simulink model "bh_4dof_LAGR_manipulator_CONTROL_DL_discrete"  (R2016b)
settings: Solver=ode23s  StartTime=0.0  StopTime=60  FixedStep=0.001  RelTol=1e-5  EnableMultiTasking=on
StopFcn:
  | bh_4dof_sim_post_process
values from neighbouring files (symbols this model uses):
  N = 3    [bh_4dof_sim_post_process.m]
undefined symbols (not defined in the file or in its folder): b1_damp, b2_damp, b3_damp, b4_damp, g, Hz, L1x, L1y, L1z, L2x, L2y, L2z, L3x, L3y, L3z, mass1, mass2, mass3, mass4, Rturn, theta1_0, theta1_dot_0, theta2_0, theta2_dot_0, theta3_0, theta3_dot_0, theta4_0, theta4_dot_0, X, Y, Z
libraries: simulink_extras x42, sm_lib x25, simulink x18, nesl_utility x17, discretizing x8
(part 1 of 4)
settings Model: Creator=bhorton  LastModifiedBy=bhorton
settings SolverCC: ZeroCrossAlgorithm=Adaptive
settings OptimizationCC: LifeSpan=inf
settings DebuggingCC: SFUnexpectedBacktrackingDiag=warning  SFNoUnconditionalDefaultTransitionDiag=warning  SFExecutionAtInitializationDiag=none
settings GRTTargetCC: TargetLangStandard=C89/C90 (ANSI)
settings ConfigComp: CovMetricSettings=dw  CovHtmlReporting=on  CovSaveCumulativeToWorkspaceVar=on  CovSaveSingleToWorkspaceVar=on  CovExternalEMLEnable=off
settings SimscapeCC: SimscapeLogDataHistory=10000  SelectedTab=General

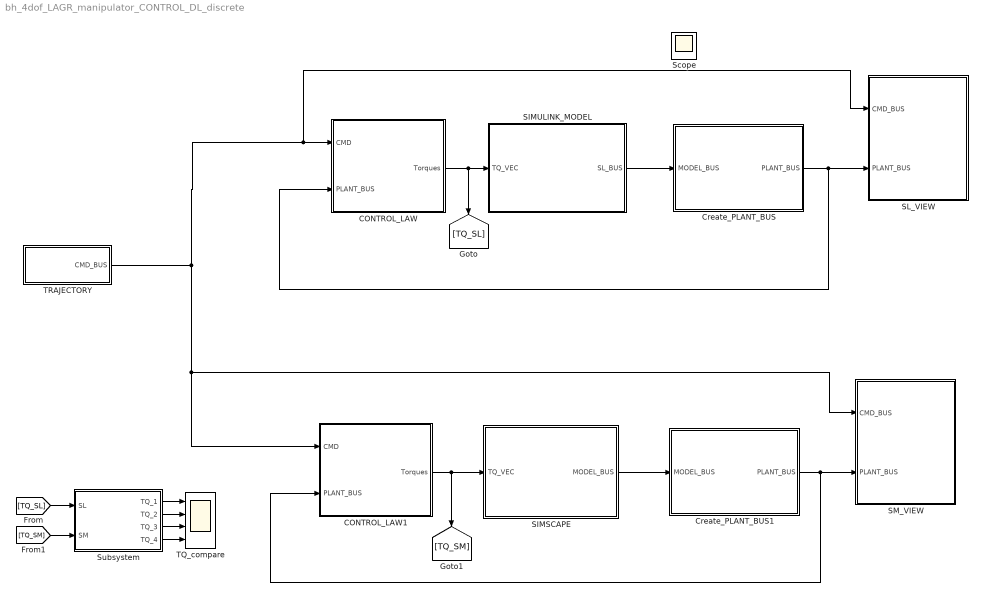
== system bh_4dof_LAGR_manipulator_CONTROL_DL_discrete ==
  CONTROL_LAW : Subsystem
  CONTROL_LAW1 : Subsystem
  Create_PLANT_BUS : Subsystem
  Create_PLANT_BUS1 : Subsystem
  SIMSCAPE : Subsystem  VariantControl=Variant
  SIMULINK_MODEL : Subsystem
  SL_VIEW : Subsystem
  SM_VIEW : Subsystem
  Subsystem : Subsystem
  TQ_compare : Scope  NumInputPorts=4
  TRAJECTORY : Subsystem
  Scope : Scope
  wires:
  TRAJECTORY/1(CMD_BUS) -> SL_VIEW/1(CMD_BUS), CONTROL_LAW/1(CMD), CONTROL_LAW1/1(CMD), SM_VIEW/1(CMD_BUS)
  Create_PLANT_BUS/1(PLANT_BUS) -> SL_VIEW/2(PLANT_BUS), CONTROL_LAW/2(PLANT_BUS)
  SIMULINK_MODEL/1(SL_BUS) -> Create_PLANT_BUS/1(MODEL_BUS)
  CONTROL_LAW/1(Torques) -> SIMULINK_MODEL/1(TQ_VEC), [TQ_SL]
  SIMSCAPE/1(MODEL_BUS) -> Create_PLANT_BUS1/1(MODEL_BUS)
  CONTROL_LAW1/1(Torques) -> SIMSCAPE/1(TQ_VEC), [TQ_SM]
  Create_PLANT_BUS1/1(PLANT_BUS) -> CONTROL_LAW1/2(PLANT_BUS), SM_VIEW/2(PLANT_BUS)
  [TQ_SL] -> Subsystem/1(SL)
  [TQ_SM] -> Subsystem/2(SM)
  Subsystem/1(TQ_1) -> TQ_compare/1
  Subsystem/4(TQ_4) -> TQ_compare/4
  Subsystem/2(TQ_2) -> TQ_compare/2
  Subsystem/3(TQ_3) -> TQ_compare/3

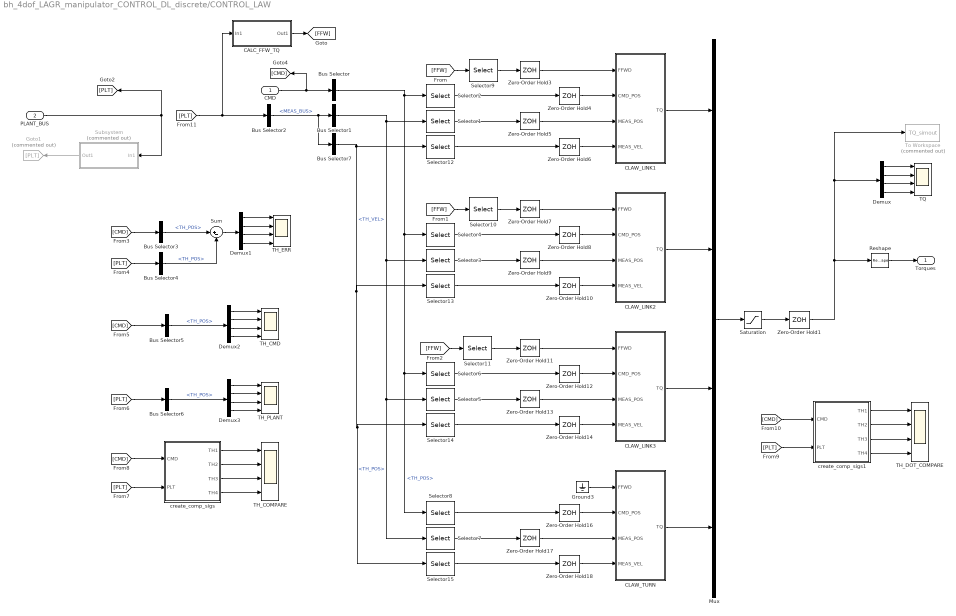
== system bh_4dof_LAGR_manipulator_CONTROL_DL_discrete/CONTROL_LAW ==
  CMD : Inport
  PLANT_BUS : Inport  Port=2
  Bus Selector{,1,3,5} (4 alike) : BusSelector  OutputSignals=TH_POS
  Bus Selector2 : BusSelector  OutputSignals=MEAS_BUS
  Bus Selector4 : BusSelector  OutputSignals=MEAS_BUS.TH_POS
  Bus Selector6 : BusSelector  OutputSignals=MEAS_BUS.TH_POS
  Bus Selector7 : BusSelector  OutputSignals=TH_VEL
  CALC_FFW_TQ : Subsystem
  CLAW_LINK1 : Subsystem
  CLAW_LINK2 : Subsystem
  CLAW_LINK3 : Subsystem
  CLAW_TURN : Subsystem
  Demux{,1..3} (4 alike) : Demux
  Goto1 : Goto  Commented=on  GotoTag=PLT
  Ground3 : Ground
  Mux : Mux
  Reshape : Reshape  OutputDimensionality=Column vector (2-D)
  Saturation : Saturate  UpperLimit=3  LowerLimit=-3
  Selector1 : Selector  InputPortWidth=4  IndexOptions=Index vector (dialog)  Indices=1  OutputSizes=1
  Selector10 : Selector  InputPortWidth=3  IndexOptions=Index vector (dialog)  Indices=2  OutputSizes=1
  Selector11 : Selector  InputPortWidth=3  IndexOptions=Index vector (dialog)  Indices=3  OutputSizes=1
  Selector12 : Selector  InputPortWidth=4  IndexOptions=Index vector (dialog)  Indices=1  OutputSizes=1
  Selector13 : Selector  InputPortWidth=4  IndexOptions=Index vector (dialog)  Indices=2  OutputSizes=1
  Selector14 : Selector  InputPortWidth=4  IndexOptions=Index vector (dialog)  Indices=3  OutputSizes=1
  Selector15 : Selector  InputPortWidth=4  IndexOptions=Index vector (dialog)  Indices=4  OutputSizes=1
  Selector2 : Selector  InputPortWidth=4  IndexOptions=Index vector (dialog)  Indices=1  OutputSizes=1
  Selector3 : Selector  InputPortWidth=4  IndexOptions=Index vector (dialog)  Indices=2  OutputSizes=1
  Selector4 : Selector  InputPortWidth=4  IndexOptions=Index vector (dialog)  Indices=2  OutputSizes=1
  Selector5 : Selector  InputPortWidth=4  IndexOptions=Index vector (dialog)  Indices=3  OutputSizes=1
  Selector6 : Selector  InputPortWidth=4  IndexOptions=Index vector (dialog)  Indices=3  OutputSizes=1
  Selector7 : Selector  InputPortWidth=4  IndexOptions=Index vector (dialog)  Indices=4  OutputSizes=1
  Selector8 : Selector  InputPortWidth=4  IndexOptions=Index vector (dialog)  Indices=4  OutputSizes=1
  Selector9 : Selector  InputPortWidth=3  IndexOptions=Index vector (dialog)  Indices=1  OutputSizes=1
  Subsystem : Subsystem  Commented=on
  Sum : Sum  Inputs=|+-
  TH_CMD : Scope  NumInputPorts=4
  TH_COMPARE : Scope  NumInputPorts=4
  TH_DOT_COMPARE : Scope  NumInputPorts=4
  TH_ERR : Scope  NumInputPorts=4
  TH_PLANT : Scope  NumInputPorts=4
  TQ : Scope  NumInputPorts=4
  To Workspace : ToWorkspace  Commented=on  VariableName=TQ_simout  SaveFormat=Structure With Time  SampleTime=-1
  Zero-Order Hold{1,3..14,16..18} (16 alike) : ZeroOrderHold  SampleTime=0.001
      settings: AttributesFormatString=DT =%<SampleTime>
  create_comp_sigs : Subsystem
  create_comp_sigs1 : Subsystem
  Torques : Outport
  wires:
  Mux/1 -> Saturation/1
  Reshape/1 -> Torques/1
  Selector9/1 -> Zero-Order Hold3/1
  CMD/1 -> [CMD], Bus Selector/1
  Selector1/1 -> Zero-Order Hold5/1
  Selector2/1 -> Zero-Order Hold4/1
  Bus Selector/1 -> Selector8/1, Selector6/1, Selector4/1, Selector2/1  "<TH_POS>"
  Bus Selector1/1 -> Selector5/1, Selector7/1, Selector3/1, Selector1/1  "<TH_POS>"
  Bus Selector2/1 -> Bus Selector7/1, Bus Selector1/1  "<MEAS_BUS>"
  Demux/1 -> TQ/1
  Demux/2 -> TQ/2
  Demux/4 -> TQ/4
  Demux/3 -> TQ/3
  CALC_FFW_TQ/1(Out1) -> [FFW]
  [FFW] -> Selector9/1
  [FFW] -> Selector10/1
  [FFW] -> Selector11/1
  Demux1/1 -> TH_ERR/1
  Demux1/2 -> TH_ERR/2
  Demux1/4 -> TH_ERR/4
  Demux1/3 -> TH_ERR/3
  PLANT_BUS/1 -> Subsystem/1(In1), [PLT]
  [CMD] -> Bus Selector3/1
  [PLT] -> Bus Selector4/1
  Bus Selector3/1 -> Sum/1  "<TH_POS>"
  Bus Selector4/1 -> Sum/2  "<TH_POS>"
  Sum/1 -> Demux1/1
  Demux2/1 -> TH_CMD/1
  Demux2/2 -> TH_CMD/2
  Demux2/4 -> TH_CMD/4
  Demux2/3 -> TH_CMD/3
  [CMD] -> Bus Selector5/1
  Bus Selector5/1 -> Demux2/1  "<TH_POS>"
  Demux3/1 -> TH_PLANT/1
  Demux3/2 -> TH_PLANT/2
  Demux3/4 -> TH_PLANT/4
  Demux3/3 -> TH_PLANT/3
  [PLT] -> Bus Selector6/1
  Bus Selector6/1 -> Demux3/1  "<TH_POS>"
  Bus Selector7/1 -> Selector15/1, Selector14/1, Selector13/1, Selector12/1  "<TH_VEL>"
  Selector12/1 -> Zero-Order Hold6/1
  CLAW_TURN/1(TQ) -> Mux/4
  CLAW_LINK3/1(TQ) -> Mux/3
  CLAW_LINK2/1(TQ) -> Mux/2
  CLAW_LINK1/1(TQ) -> Mux/1
  Saturation/1 -> Zero-Order Hold1/1
  Zero-Order Hold3/1 -> CLAW_LINK1/1(FFWD)
  Zero-Order Hold4/1 -> CLAW_LINK1/2(CMD_POS)
  Zero-Order Hold5/1 -> CLAW_LINK1/3(MEAS_POS)
  Zero-Order Hold6/1 -> CLAW_LINK1/4(MEAS_VEL)
  Selector10/1 -> Zero-Order Hold7/1
  Selector3/1 -> Zero-Order Hold9/1
  Selector4/1 -> Zero-Order Hold8/1
  Selector13/1 -> Zero-Order Hold10/1
  Zero-Order Hold7/1 -> CLAW_LINK2/1(FFWD)
  Zero-Order Hold8/1 -> CLAW_LINK2/2(CMD_POS)
  Zero-Order Hold9/1 -> CLAW_LINK2/3(MEAS_POS)
  Zero-Order Hold10/1 -> CLAW_LINK2/4(MEAS_VEL)
  Selector5/1 -> Zero-Order Hold13/1
  Selector6/1 -> Zero-Order Hold12/1
  Selector14/1 -> Zero-Order Hold14/1
  Zero-Order Hold11/1 -> CLAW_LINK3/1(FFWD)
  Zero-Order Hold12/1 -> CLAW_LINK3/2(CMD_POS)
  Zero-Order Hold13/1 -> CLAW_LINK3/3(MEAS_POS)
  Zero-Order Hold14/1 -> CLAW_LINK3/4(MEAS_VEL)
  Selector11/1 -> Zero-Order Hold11/1
  Selector7/1 -> Zero-Order Hold17/1
  Selector8/1 -> Zero-Order Hold16/1
  Selector15/1 -> Zero-Order Hold18/1
  Zero-Order Hold16/1 -> CLAW_TURN/2(CMD_POS)
  Zero-Order Hold17/1 -> CLAW_TURN/3(MEAS_POS)
  Zero-Order Hold18/1 -> CLAW_TURN/4(MEAS_VEL)
  Ground3/1 -> CLAW_TURN/1(FFWD)
  [PLT] -> create_comp_sigs/2(PLT)
  [CMD] -> create_comp_sigs/1(CMD)
  create_comp_sigs/1(TH1) -> TH_COMPARE/1
  create_comp_sigs/2(TH2) -> TH_COMPARE/2
  create_comp_sigs/3(TH3) -> TH_COMPARE/3
  create_comp_sigs/4(TH4) -> TH_COMPARE/4
  [PLT] -> create_comp_sigs1/2(PLT)
  [CMD] -> create_comp_sigs1/1(CMD)
  create_comp_sigs1/1(TH1) -> TH_DOT_COMPARE/1
  create_comp_sigs1/2(TH2) -> TH_DOT_COMPARE/2
  create_comp_sigs1/3(TH3) -> TH_DOT_COMPARE/3
  create_comp_sigs1/4(TH4) -> TH_DOT_COMPARE/4
  Zero-Order Hold1/1 -> Reshape/1, To Workspace/1, Demux/1
  Subsystem/1(Out1) -> Goto1/1
  [PLT] -> CALC_FFW_TQ/1(In1), Bus Selector2/1

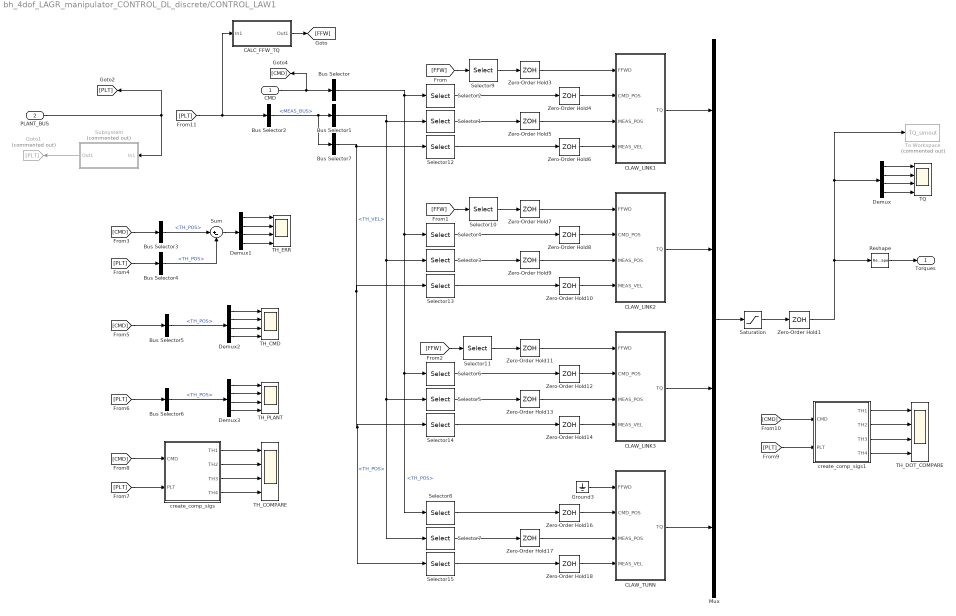
== system bh_4dof_LAGR_manipulator_CONTROL_DL_discrete/CONTROL_LAW1 ==
  CMD : Inport
  PLANT_BUS : Inport  Port=2
  Bus Selector{,1,3,5} (4 alike) : BusSelector  OutputSignals=TH_POS
  Bus Selector2 : BusSelector  OutputSignals=MEAS_BUS
  Bus Selector4 : BusSelector  OutputSignals=MEAS_BUS.TH_POS
  Bus Selector6 : BusSelector  OutputSignals=MEAS_BUS.TH_POS
  Bus Selector7 : BusSelector  OutputSignals=TH_VEL
  CALC_FFW_TQ : Subsystem
  CLAW_LINK1 : Subsystem
  CLAW_LINK2 : Subsystem
  CLAW_LINK3 : Subsystem
  CLAW_TURN : Subsystem
  Demux{,1..3} (4 alike) : Demux
  Goto1 : Goto  Commented=on  GotoTag=PLT
  Ground3 : Ground
  Mux : Mux
  Reshape : Reshape  OutputDimensionality=Column vector (2-D)
  Saturation : Saturate  UpperLimit=3  LowerLimit=-3
  Selector1 : Selector  InputPortWidth=4  IndexOptions=Index vector (dialog)  Indices=1  OutputSizes=1
  Selector10 : Selector  InputPortWidth=3  IndexOptions=Index vector (dialog)  Indices=2  OutputSizes=1
  Selector11 : Selector  InputPortWidth=3  IndexOptions=Index vector (dialog)  Indices=3  OutputSizes=1
  Selector12 : Selector  InputPortWidth=4  IndexOptions=Index vector (dialog)  Indices=1  OutputSizes=1
  Selector13 : Selector  InputPortWidth=4  IndexOptions=Index vector (dialog)  Indices=2  OutputSizes=1
  Selector14 : Selector  InputPortWidth=4  IndexOptions=Index vector (dialog)  Indices=3  OutputSizes=1
  Selector15 : Selector  InputPortWidth=4  IndexOptions=Index vector (dialog)  Indices=4  OutputSizes=1
  Selector2 : Selector  InputPortWidth=4  IndexOptions=Index vector (dialog)  Indices=1  OutputSizes=1
  Selector3 : Selector  InputPortWidth=4  IndexOptions=Index vector (dialog)  Indices=2  OutputSizes=1
  Selector4 : Selector  InputPortWidth=4  IndexOptions=Index vector (dialog)  Indices=2  OutputSizes=1
  Selector5 : Selector  InputPortWidth=4  IndexOptions=Index vector (dialog)  Indices=3  OutputSizes=1
  Selector6 : Selector  InputPortWidth=4  IndexOptions=Index vector (dialog)  Indices=3  OutputSizes=1
  Selector7 : Selector  InputPortWidth=4  IndexOptions=Index vector (dialog)  Indices=4  OutputSizes=1
  Selector8 : Selector  InputPortWidth=4  IndexOptions=Index vector (dialog)  Indices=4  OutputSizes=1
  Selector9 : Selector  InputPortWidth=3  IndexOptions=Index vector (dialog)  Indices=1  OutputSizes=1
  Subsystem : Subsystem  Commented=on
  Sum : Sum  Inputs=|+-
  TH_CMD : Scope  NumInputPorts=4
  TH_COMPARE : Scope  NumInputPorts=4
  TH_DOT_COMPARE : Scope  NumInputPorts=4
  TH_ERR : Scope  NumInputPorts=4
  TH_PLANT : Scope  NumInputPorts=4
  TQ : Scope  NumInputPorts=4
  To Workspace : ToWorkspace  Commented=on  VariableName=TQ_simout  SaveFormat=Structure With Time  SampleTime=-1
  Zero-Order Hold{1,3..14,16..18} (16 alike) : ZeroOrderHold  SampleTime=0.001
      settings: AttributesFormatString=DT =%<SampleTime>
  create_comp_sigs : Subsystem
  create_comp_sigs1 : Subsystem
  Torques : Outport
  wires:
  Mux/1 -> Saturation/1
  Reshape/1 -> Torques/1
  Selector9/1 -> Zero-Order Hold3/1
  CMD/1 -> [CMD], Bus Selector/1
  Selector1/1 -> Zero-Order Hold5/1
  Selector2/1 -> Zero-Order Hold4/1
  Bus Selector/1 -> Selector8/1, Selector6/1, Selector4/1, Selector2/1  "<TH_POS>"
  Bus Selector1/1 -> Selector5/1, Selector7/1, Selector3/1, Selector1/1  "<TH_POS>"
  Bus Selector2/1 -> Bus Selector7/1, Bus Selector1/1  "<MEAS_BUS>"
  Demux/1 -> TQ/1
  Demux/2 -> TQ/2
  Demux/4 -> TQ/4
  Demux/3 -> TQ/3
  CALC_FFW_TQ/1(Out1) -> [FFW]
  [FFW] -> Selector9/1
  [FFW] -> Selector10/1
  [FFW] -> Selector11/1
  Demux1/1 -> TH_ERR/1
  Demux1/2 -> TH_ERR/2
  Demux1/4 -> TH_ERR/4
  Demux1/3 -> TH_ERR/3
  PLANT_BUS/1 -> Subsystem/1(In1), [PLT]
  [CMD] -> Bus Selector3/1
  [PLT] -> Bus Selector4/1
  Bus Selector3/1 -> Sum/1  "<TH_POS>"
  Bus Selector4/1 -> Sum/2  "<TH_POS>"
  Sum/1 -> Demux1/1
  Demux2/1 -> TH_CMD/1
  Demux2/2 -> TH_CMD/2
  Demux2/4 -> TH_CMD/4
  Demux2/3 -> TH_CMD/3
  [CMD] -> Bus Selector5/1
  Bus Selector5/1 -> Demux2/1  "<TH_POS>"
  Demux3/1 -> TH_PLANT/1
  Demux3/2 -> TH_PLANT/2
  Demux3/4 -> TH_PLANT/4
  Demux3/3 -> TH_PLANT/3
  [PLT] -> Bus Selector6/1
  Bus Selector6/1 -> Demux3/1  "<TH_POS>"
  Bus Selector7/1 -> Selector15/1, Selector14/1, Selector13/1, Selector12/1  "<TH_VEL>"
  Selector12/1 -> Zero-Order Hold6/1
  CLAW_TURN/1(TQ) -> Mux/4
  CLAW_LINK3/1(TQ) -> Mux/3
  CLAW_LINK2/1(TQ) -> Mux/2
  CLAW_LINK1/1(TQ) -> Mux/1
  Saturation/1 -> Zero-Order Hold1/1
  Zero-Order Hold3/1 -> CLAW_LINK1/1(FFWD)
  Zero-Order Hold4/1 -> CLAW_LINK1/2(CMD_POS)
  Zero-Order Hold5/1 -> CLAW_LINK1/3(MEAS_POS)
  Zero-Order Hold6/1 -> CLAW_LINK1/4(MEAS_VEL)
  Selector10/1 -> Zero-Order Hold7/1
  Selector3/1 -> Zero-Order Hold9/1
  Selector4/1 -> Zero-Order Hold8/1
  Selector13/1 -> Zero-Order Hold10/1
  Zero-Order Hold7/1 -> CLAW_LINK2/1(FFWD)
  Zero-Order Hold8/1 -> CLAW_LINK2/2(CMD_POS)
  Zero-Order Hold9/1 -> CLAW_LINK2/3(MEAS_POS)
  Zero-Order Hold10/1 -> CLAW_LINK2/4(MEAS_VEL)
  Selector5/1 -> Zero-Order Hold13/1
  Selector6/1 -> Zero-Order Hold12/1
  Selector14/1 -> Zero-Order Hold14/1
  Zero-Order Hold11/1 -> CLAW_LINK3/1(FFWD)
  Zero-Order Hold12/1 -> CLAW_LINK3/2(CMD_POS)
  Zero-Order Hold13/1 -> CLAW_LINK3/3(MEAS_POS)
  Zero-Order Hold14/1 -> CLAW_LINK3/4(MEAS_VEL)
  Selector11/1 -> Zero-Order Hold11/1
  Selector7/1 -> Zero-Order Hold17/1
  Selector8/1 -> Zero-Order Hold16/1
  Selector15/1 -> Zero-Order Hold18/1
  Zero-Order Hold16/1 -> CLAW_TURN/2(CMD_POS)
  Zero-Order Hold17/1 -> CLAW_TURN/3(MEAS_POS)
  Zero-Order Hold18/1 -> CLAW_TURN/4(MEAS_VEL)
  Ground3/1 -> CLAW_TURN/1(FFWD)
  [PLT] -> create_comp_sigs/2(PLT)
  [CMD] -> create_comp_sigs/1(CMD)
  create_comp_sigs/1(TH1) -> TH_COMPARE/1
  create_comp_sigs/2(TH2) -> TH_COMPARE/2
  create_comp_sigs/3(TH3) -> TH_COMPARE/3
  create_comp_sigs/4(TH4) -> TH_COMPARE/4
  [PLT] -> create_comp_sigs1/2(PLT)
  [CMD] -> create_comp_sigs1/1(CMD)
  create_comp_sigs1/1(TH1) -> TH_DOT_COMPARE/1
  create_comp_sigs1/2(TH2) -> TH_DOT_COMPARE/2
  create_comp_sigs1/3(TH3) -> TH_DOT_COMPARE/3
  create_comp_sigs1/4(TH4) -> TH_DOT_COMPARE/4
  Zero-Order Hold1/1 -> Reshape/1, To Workspace/1, Demux/1
  Subsystem/1(Out1) -> Goto1/1
  [PLT] -> CALC_FFW_TQ/1(In1), Bus Selector2/1

== system bh_4dof_LAGR_manipulator_CONTROL_DL_discrete/Create_PLANT_BUS ==
  MODEL_BUS : Inport
  CALC_BUS : Subsystem
  MEAS : Subsystem
  Subsystem : Subsystem
  Subsystem1 : Subsystem
  PLANT_BUS : Outport
  wires:
  MODEL_BUS/1 -> MEAS/1(MODEL_BUS), CALC_BUS/1(MODEL_BUS), Subsystem/1(MODEL)
  Subsystem/1(PLANT_B) -> PLANT_BUS/1
  CALC_BUS/1(CALC_POS) -> Subsystem1/1(POS), Subsystem/3(CALC_POS)
  MEAS/1(MEAS) -> Subsystem/2(MEAS)
  Subsystem1/1(GTQ) -> Subsystem/4(CALC_GRAV_TQ)

== system bh_4dof_LAGR_manipulator_CONTROL_DL_discrete/Create_PLANT_BUS1 ==
  MODEL_BUS : Inport
  CALC_BUS : Subsystem
  MEAS : Subsystem
  Subsystem : Subsystem
  Subsystem1 : Subsystem
  PLANT_BUS : Outport
  wires:
  MODEL_BUS/1 -> MEAS/1(MODEL_BUS), CALC_BUS/1(MODEL_BUS), Subsystem/1(MODEL)
  Subsystem/1(PLANT_B) -> PLANT_BUS/1
  CALC_BUS/1(CALC_POS) -> Subsystem1/1(POS), Subsystem/3(CALC_POS)
  MEAS/1(MEAS) -> Subsystem/2(MEAS)
  Subsystem1/1(GTQ) -> Subsystem/4(CALC_GRAV_TQ)

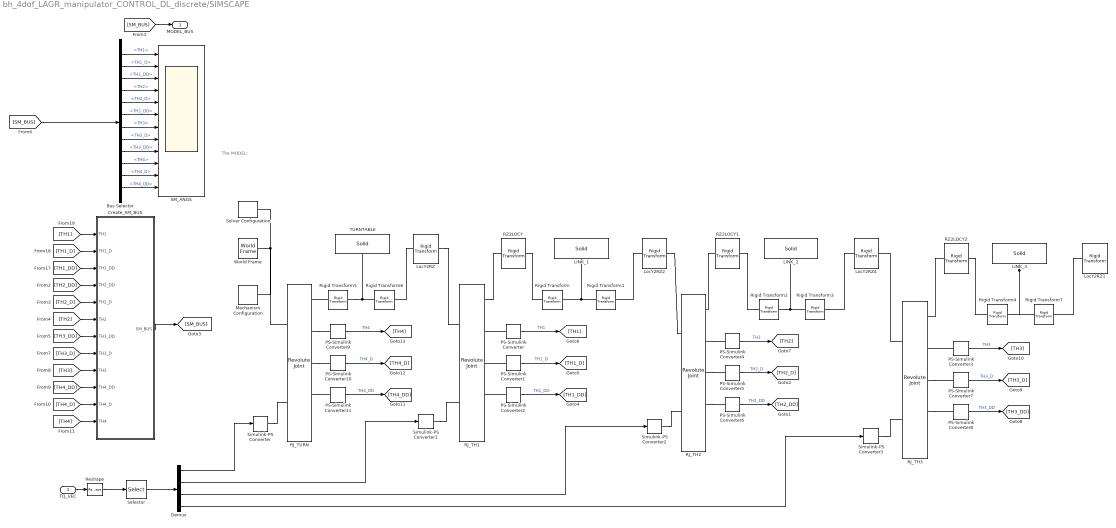
== system bh_4dof_LAGR_manipulator_CONTROL_DL_discrete/SIMSCAPE ==
  note: The MODEL:
  TQ_VEC : Inport
  Bus Selector : BusSelector  OutputSignals=TH1,TH1_D,TH1_DD,TH2,TH2_D,TH2_DD,TH3,TH3_D,TH3_DD,TH4,TH4_D,TH4_DD
  Create_SM_BUS : Subsystem
  Demux : Demux
  LINK_1 : sm_lib/Body Elements/Solid  InertiaType=CalculateFromGeometry  Mass=1  MassUnits=kg  CenterOfMass=[0 0 0]  CenterOfMassUnits=m  MomentsOfInertia=[1 1 1]  MomentsOfInertiaUnits=kg*m^2  ProductsOfInertia=[0 0 0]  ProductsOfInertiaUnits=kg*m^2  DensityBased=on  Density=density  DensityUnits=kg/(m^3)  DoExposeReferenceFrame=on  SerializedFrames=<Frames/>  GraphicType=FromGeometry  MarkerShape=Sphere  MarkerSize=10  GraphicVisPropType=SimpleVisualProperties  GraphicDiffuseColor=[0.2 0.2 1.0]  GraphicSpecularColor=[0.5 0.5 0.5 1.0]  GraphicAmbientColor=[0.15 0.15 0.15 1.0]  GraphicEmissiveColor=[0.0 0.0 0.0 1.0]  GraphicShininess=75  GraphicOpacity=1.0  GeometryShape=Brick  RectangleSize=[1 1]  RectangleSizeUnits=m  BrickDimensions=[L1x, L1y, L1z ]  BrickDimensionUnits=m  CylinderRadius=1  CylinderRadiusUnits=m  CylinderLength=1  CylinderLengthUnits=m  SphereRadius=1  SphereRadiusUnits=m  EllipsoidRadii=[1 1 1]  EllipsoidRadiiUnits=m  ExtrusionCrossSection=[1 1; -1 1; -1 -1; 1 -1]  ExtrusionCrossSectionUnits=m  ExtrusionLength=1  ExtrusionLengthUnits=m  PolygonNumSides=3  PolygonOuterRadius=1  PolygonOuterRadiusUnits=m  ExtGeomFileType=STEP  ExtGeomFileUnits=m  RevolutionCrossSection=[1 1; 1 -1; 2 -1; 2 1]  RevolutionCrossSectionUnits=m  RevolutionExtent=Full  RevolutionAngle=180  RevolutionAngleUnits=deg
  LINK_2 : sm_lib/Body Elements/Solid  InertiaType=CalculateFromGeometry  Mass=1  MassUnits=kg  CenterOfMass=[0 0 0]  CenterOfMassUnits=m  MomentsOfInertia=[1 1 1]  MomentsOfInertiaUnits=kg*m^2  ProductsOfInertia=[0 0 0]  ProductsOfInertiaUnits=kg*m^2  DensityBased=on  Density=density  DensityUnits=kg/(m^3)  DoExposeReferenceFrame=on  SerializedFrames=<Frames/>  GraphicType=FromGeometry  MarkerShape=Sphere  MarkerSize=10  GraphicVisPropType=SimpleVisualProperties  GraphicDiffuseColor=[0.8 0.8 1.0]  GraphicSpecularColor=[0.5 0.5 0.5 1.0]  GraphicAmbientColor=[0.15 0.15 0.15 1.0]  GraphicEmissiveColor=[0.0 0.0 0.0 1.0]  GraphicShininess=75  GraphicOpacity=1.0  GeometryShape=Brick  RectangleSize=[1 1]  RectangleSizeUnits=m  BrickDimensions=[L2x, L2y, L2z ]  BrickDimensionUnits=m  CylinderRadius=1  CylinderRadiusUnits=m  CylinderLength=1  CylinderLengthUnits=m  SphereRadius=1  SphereRadiusUnits=m  EllipsoidRadii=[1 1 1]  EllipsoidRadiiUnits=m  ExtrusionCrossSection=[1 1; -1 1; -1 -1; 1 -1]  ExtrusionCrossSectionUnits=m  ExtrusionLength=1  ExtrusionLengthUnits=m  PolygonNumSides=3  PolygonOuterRadius=1  PolygonOuterRadiusUnits=m  ExtGeomFileType=STEP  ExtGeomFileUnits=m  RevolutionCrossSection=[1 1; 1 -1; 2 -1; 2 1]  RevolutionCrossSectionUnits=m  RevolutionExtent=Full  RevolutionAngle=180  RevolutionAngleUnits=deg
  LINK_3 : sm_lib/Body Elements/Solid  InertiaType=CalculateFromGeometry  Mass=1  MassUnits=kg  CenterOfMass=[0 0 0]  CenterOfMassUnits=m  MomentsOfInertia=[1 1 1]  MomentsOfInertiaUnits=kg*m^2  ProductsOfInertia=[0 0 0]  ProductsOfInertiaUnits=kg*m^2  DensityBased=on  Density=density  DensityUnits=kg/(m^3)  DoExposeReferenceFrame=on  SerializedFrames=<Frames/>  GraphicType=FromGeometry  MarkerShape=Sphere  MarkerSize=10  GraphicVisPropType=SimpleVisualProperties  GraphicDiffuseColor=[1.0 0.8 0.4]  GraphicSpecularColor=[0.5 0.5 0.5 1.0]  GraphicAmbientColor=[0.15 0.15 0.15 1.0]  GraphicEmissiveColor=[0.0 0.0 0.0 1.0]  GraphicShininess=75  GraphicOpacity=1.0  GeometryShape=Brick  RectangleSize=[1 1]  RectangleSizeUnits=m  BrickDimensions=[L3x, L3y, L3z ]  BrickDimensionUnits=m  CylinderRadius=1  CylinderRadiusUnits=m  CylinderLength=1  CylinderLengthUnits=m  SphereRadius=1  SphereRadiusUnits=m  EllipsoidRadii=[1 1 1]  EllipsoidRadiiUnits=m  ExtrusionCrossSection=[1 1; -1 1; -1 -1; 1 -1]  ExtrusionCrossSectionUnits=m  ExtrusionLength=1  ExtrusionLengthUnits=m  PolygonNumSides=3  PolygonOuterRadius=1  PolygonOuterRadiusUnits=m  ExtGeomFileType=STEP  ExtGeomFileUnits=m  RevolutionCrossSection=[1 1; 1 -1; 2 -1; 2 1]  RevolutionCrossSectionUnits=m  RevolutionExtent=Full  RevolutionAngle=180  RevolutionAngleUnits=deg
  LocY2RZ{,1..2,4} (4 alike) : sm_lib/Frames and Transforms/Rigid Transform  TranslationMethod=None  TranslationStandardOffset=Hz/2  TranslationLengthUnit=m  TranslationStandardAxis=+Z  TranslationCartesianOffset=[0 0 0]  TranslationROffset=0  TranslationROffsetUnits=m  TranslationZOffset=0  TranslationZOffsetUnits=m  TranslationThetaOffset=0  TranslationThetaOffsetUnits=deg  RotationMethod=AlignedAxes  RotationAngleUnits=deg  RotationStandardAxis=+Z  RotationAngle=0.0  RotationArbitraryAxis=[0 0 1]  FollAlignAxisA=+X  BaseAlignAxisA=+Y  FollAlignAxisB=+Y  BaseAlignAxisB=+Z  RotationSequenceAxes=FollowerAxes  RotationSequence=XYX  RotationSequenceAngles=[0 0 0]  RotationSequenceAnglesUnits=deg  RotationMatrix=[1 0 0; 0 1 0; 0 0 1]
  Mechanism Configuration : sm_lib/Utilities/Mechanism Configuration  UniformGravity=Constant  GravityVector=[0 0 -9.80665 ]  GravityUnits=m/s^2  LinearizationDelta=1e-4
  PS-Simulink Converter{,3..4,9} (4 alike) : nesl_utility/PS-Simulink Converter  PhysicalDomain=network_engine_domain  SubClassName=ps_output  LeftPortType=input  RightPortType=output  PseudoPeriodic=off  Frequencies=[]  Unit=rad  AffineConversion=off
  PS-Simulink Converter{1,5,7,10} (4 alike) : nesl_utility/PS-Simulink Converter  PhysicalDomain=network_engine_domain  SubClassName=ps_output  LeftPortType=input  RightPortType=output  PseudoPeriodic=off  Frequencies=[]  Unit=rad/s  AffineConversion=off
  PS-Simulink Converter{2,6,8,11} (4 alike) : nesl_utility/PS-Simulink Converter  PhysicalDomain=network_engine_domain  SubClassName=ps_output  LeftPortType=input  RightPortType=output  PseudoPeriodic=off  Frequencies=[]  Unit=rad/s^2  AffineConversion=off
  RJ_TH1 : sm_lib/Joints/Revolute Joint  SenseConstraintForce=on  SenseConstraintForceX=off  SenseConstraintForceY=off  SenseConstraintForceZ=off  SenseConstraintTorque=off  SenseConstraintTorqueX=off  SenseConstraintTorqueY=off  SenseConstraintTorqueZ=off  SenseTotalForce=off  SenseTotalForceX=off  SenseTotalForceY=off  SenseTotalForceZ=off  SenseTotalTorque=off  SenseTotalTorqueX=off  SenseTotalTorqueY=off  SenseTotalTorqueZ=off  CompositeWrenchDir=BaseOnFollower  CompositeWrenchFrame=BaseFrame  EquilibriumPosition=0  EquilibriumPositionUnits=deg  SpringStiffness=0  SpringStiffnessUnits=N*m/deg  DampingCoefficient=b1_damp  DampingCoefficientUnits=N*m/(rad/s)  TorqueActuationMode=InputTorque  MotionActuationMode=ComputedMotion  SensePosition=on  SenseVelocity=on  SenseAcceleration=on  SenseTorqueForce=off  PositionTargetSpecify=on  PositionTargetPriority=Low  PositionTargetValue=theta1_0  PositionTargetValueUnits=rad  VelocityTargetSpecify=on  VelocityTargetPriority=High  VelocityTargetValue=theta1_dot_0  VelocityTargetValueUnits=rad/s
      settings: AttributesFormatString=|
      | %<DampingCoefficient>
      | %<PositionTargetValue>
      | %<VelocityTargetValue>
  RJ_TH2 : sm_lib/Joints/Revolute Joint  SenseConstraintForce=on  SenseConstraintForceX=off  SenseConstraintForceY=off  SenseConstraintForceZ=off  SenseConstraintTorque=off  SenseConstraintTorqueX=off  SenseConstraintTorqueY=off  SenseConstraintTorqueZ=off  SenseTotalForce=off  SenseTotalForceX=off  SenseTotalForceY=off  SenseTotalForceZ=off  SenseTotalTorque=off  SenseTotalTorqueX=off  SenseTotalTorqueY=off  SenseTotalTorqueZ=off  CompositeWrenchDir=BaseOnFollower  CompositeWrenchFrame=BaseFrame  EquilibriumPosition=0  EquilibriumPositionUnits=deg  SpringStiffness=0  SpringStiffnessUnits=N*m/deg  DampingCoefficient=b2_damp  DampingCoefficientUnits=N*m/(rad/s)  TorqueActuationMode=InputTorque  MotionActuationMode=ComputedMotion  SensePosition=on  SenseVelocity=on  SenseAcceleration=on  SenseTorqueForce=off  PositionTargetSpecify=on  PositionTargetPriority=Low  PositionTargetValue=theta2_0  PositionTargetValueUnits=rad  VelocityTargetSpecify=on  VelocityTargetPriority=High  VelocityTargetValue=theta2_dot_0  VelocityTargetValueUnits=rad/s
      settings: AttributesFormatString=|
      | %<DampingCoefficient>
      | %<PositionTargetValue>
      | %<VelocityTargetValue>
  RJ_TH3 : sm_lib/Joints/Revolute Joint  SenseConstraintForce=on  SenseConstraintForceX=off  SenseConstraintForceY=off  SenseConstraintForceZ=off  SenseConstraintTorque=off  SenseConstraintTorqueX=off  SenseConstraintTorqueY=off  SenseConstraintTorqueZ=off  SenseTotalForce=off  SenseTotalForceX=off  SenseTotalForceY=off  SenseTotalForceZ=off  SenseTotalTorque=off  SenseTotalTorqueX=off  SenseTotalTorqueY=off  SenseTotalTorqueZ=off  CompositeWrenchDir=BaseOnFollower  CompositeWrenchFrame=BaseFrame  EquilibriumPosition=0  EquilibriumPositionUnits=deg  SpringStiffness=0  SpringStiffnessUnits=N*m/deg  DampingCoefficient=b3_damp  DampingCoefficientUnits=N*m/(rad/s)  TorqueActuationMode=InputTorque  MotionActuationMode=ComputedMotion  SensePosition=on  SenseVelocity=on  SenseAcceleration=on  SenseTorqueForce=off  PositionTargetSpecify=on  PositionTargetPriority=Low  PositionTargetValue=theta3_0  PositionTargetValueUnits=rad  VelocityTargetSpecify=on  VelocityTargetPriority=High  VelocityTargetValue=theta3_dot_0  VelocityTargetValueUnits=rad/s
      settings: AttributesFormatString=|
      | %<DampingCoefficient>
      | %<PositionTargetValue>
      | %<VelocityTargetValue>
  RJ_TURN : sm_lib/Joints/Revolute Joint  SenseConstraintForce=on  SenseConstraintForceX=off  SenseConstraintForceY=off  SenseConstraintForceZ=off  SenseConstraintTorque=off  SenseConstraintTorqueX=off  SenseConstraintTorqueY=off  SenseConstraintTorqueZ=off  SenseTotalForce=off  SenseTotalForceX=off  SenseTotalForceY=off  SenseTotalForceZ=off  SenseTotalTorque=off  SenseTotalTorqueX=off  SenseTotalTorqueY=off  SenseTotalTorqueZ=off  CompositeWrenchDir=BaseOnFollower  CompositeWrenchFrame=BaseFrame  EquilibriumPosition=0  EquilibriumPositionUnits=deg  SpringStiffness=0  SpringStiffnessUnits=N*m/deg  DampingCoefficient=b4_damp  DampingCoefficientUnits=N*m/(rad/s)  TorqueActuationMode=InputTorque  MotionActuationMode=ComputedMotion  SensePosition=on  SenseVelocity=on  SenseAcceleration=on  SenseTorqueForce=off  PositionTargetSpecify=on  PositionTargetPriority=Low  PositionTargetValue=theta4_0  PositionTargetValueUnits=rad  VelocityTargetSpecify=on  VelocityTargetPriority=High  VelocityTargetValue=theta4_dot_0  VelocityTargetValueUnits=rad/s
      settings: AttributesFormatString=|
      | %<DampingCoefficient>
      | %<PositionTargetValue>
      | %<VelocityTargetValue>
  RZ2LOCY : sm_lib/Frames and Transforms/Rigid Transform  TranslationMethod=None  TranslationStandardOffset=Hz/2  TranslationLengthUnit=m  TranslationStandardAxis=+Z  TranslationCartesianOffset=[0 0 0]  TranslationROffset=0  TranslationROffsetUnits=m  TranslationZOffset=0  TranslationZOffsetUnits=m  TranslationThetaOffset=0  TranslationThetaOffsetUnits=deg  RotationMethod=AlignedAxes  RotationAngleUnits=deg  RotationStandardAxis=+Z  RotationAngle=0.0  RotationArbitraryAxis=[0 0 1]  FollAlignAxisA=+Y  BaseAlignAxisA=+X  FollAlignAxisB=+X  BaseAlignAxisB=+Z  RotationSequenceAxes=FollowerAxes  RotationSequence=XYX  RotationSequenceAngles=[0 0 0]  RotationSequenceAnglesUnits=deg  RotationMatrix=[1 0 0; 0 1 0; 0 0 1]
  RZ2LOCY1 : sm_lib/Frames and Transforms/Rigid Transform  TranslationMethod=None  TranslationStandardOffset=Hz/2  TranslationLengthUnit=m  TranslationStandardAxis=+Z  TranslationCartesianOffset=[0 0 0]  TranslationROffset=0  TranslationROffsetUnits=m  TranslationZOffset=0  TranslationZOffsetUnits=m  TranslationThetaOffset=0  TranslationThetaOffsetUnits=deg  RotationMethod=AlignedAxes  RotationAngleUnits=deg  RotationStandardAxis=+Z  RotationAngle=0.0  RotationArbitraryAxis=[0 0 1]  FollAlignAxisA=+Y  BaseAlignAxisA=+X  FollAlignAxisB=+X  BaseAlignAxisB=+Z  RotationSequenceAxes=FollowerAxes  RotationSequence=XYX  RotationSequenceAngles=[0 0 0]  RotationSequenceAnglesUnits=deg  RotationMatrix=[1 0 0; 0 1 0; 0 0 1]
  RZ2LOCY2 : sm_lib/Frames and Transforms/Rigid Transform  TranslationMethod=None  TranslationStandardOffset=Hz/2  TranslationLengthUnit=m  TranslationStandardAxis=+Z  TranslationCartesianOffset=[0 0 0]  TranslationROffset=0  TranslationROffsetUnits=m  TranslationZOffset=0  TranslationZOffsetUnits=m  TranslationThetaOffset=0  TranslationThetaOffsetUnits=deg  RotationMethod=AlignedAxes  RotationAngleUnits=deg  RotationStandardAxis=+Z  RotationAngle=0.0  RotationArbitraryAxis=[0 0 1]  FollAlignAxisA=+Y  BaseAlignAxisA=+X  FollAlignAxisB=+X  BaseAlignAxisB=+Z  RotationSequenceAxes=FollowerAxes  RotationSequence=XYX  RotationSequenceAngles=[0 0 0]  RotationSequenceAnglesUnits=deg  RotationMatrix=[1 0 0; 0 1 0; 0 0 1]
  Reshape : Reshape  OutputDimensionality=Column vector (2-D)
  Rigid Transform : sm_lib/Frames and Transforms/Rigid Transform  TranslationMethod=StandardAxis  TranslationStandardOffset=L1y/2  TranslationLengthUnit=m  TranslationStandardAxis=+Y  TranslationCartesianOffset=[0 0 0]  TranslationROffset=0  TranslationROffsetUnits=m  TranslationZOffset=0  TranslationZOffsetUnits=m  TranslationThetaOffset=0  TranslationThetaOffsetUnits=deg  RotationMethod=None  RotationAngleUnits=deg  RotationStandardAxis=+Z  RotationAngle=0.0  RotationArbitraryAxis=[0 0 1]  FollAlignAxisA=+X  BaseAlignAxisA=+Y  FollAlignAxisB=+Y  BaseAlignAxisB=+Z  RotationSequenceAxes=FollowerAxes  RotationSequence=XYX  RotationSequenceAngles=[0 0 0]  RotationSequenceAnglesUnits=deg  RotationMatrix=[1 0 0; 0 1 0; 0 0 1]
  Rigid Transform1 : sm_lib/Frames and Transforms/Rigid Transform  TranslationMethod=StandardAxis  TranslationStandardOffset=L1y/2  TranslationLengthUnit=m  TranslationStandardAxis=+Y  TranslationCartesianOffset=[0 0 0]  TranslationROffset=0  TranslationROffsetUnits=m  TranslationZOffset=0  TranslationZOffsetUnits=m  TranslationThetaOffset=0  TranslationThetaOffsetUnits=deg  RotationMethod=None  RotationAngleUnits=deg  RotationStandardAxis=+Z  RotationAngle=0.0  RotationArbitraryAxis=[0 0 1]  FollAlignAxisA=+X  BaseAlignAxisA=+Y  FollAlignAxisB=+Y  BaseAlignAxisB=+Z  RotationSequenceAxes=FollowerAxes  RotationSequence=XYX  RotationSequenceAngles=[0 0 0]  RotationSequenceAnglesUnits=deg  RotationMatrix=[1 0 0; 0 1 0; 0 0 1]
  Rigid Transform2 : sm_lib/Frames and Transforms/Rigid Transform  TranslationMethod=StandardAxis  TranslationStandardOffset=L2y/2  TranslationLengthUnit=m  TranslationStandardAxis=+Y  TranslationCartesianOffset=[0 0 0]  TranslationROffset=0  TranslationROffsetUnits=m  TranslationZOffset=0  TranslationZOffsetUnits=m  TranslationThetaOffset=0  TranslationThetaOffsetUnits=deg  RotationMethod=None  RotationAngleUnits=deg  RotationStandardAxis=+Z  RotationAngle=0.0  RotationArbitraryAxis=[0 0 1]  FollAlignAxisA=+X  BaseAlignAxisA=+Y  FollAlignAxisB=+Y  BaseAlignAxisB=+Z  RotationSequenceAxes=FollowerAxes  RotationSequence=XYX  RotationSequenceAngles=[0 0 0]  RotationSequenceAnglesUnits=deg  RotationMatrix=[1 0 0; 0 1 0; 0 0 1]
  Rigid Transform3 : sm_lib/Frames and Transforms/Rigid Transform  TranslationMethod=StandardAxis  TranslationStandardOffset=L2y/2  TranslationLengthUnit=m  TranslationStandardAxis=+Y  TranslationCartesianOffset=[0 0 0]  TranslationROffset=0  TranslationROffsetUnits=m  TranslationZOffset=0  TranslationZOffsetUnits=m  TranslationThetaOffset=0  TranslationThetaOffsetUnits=deg  RotationMethod=None  RotationAngleUnits=deg  RotationStandardAxis=+Z  RotationAngle=0.0  RotationArbitraryAxis=[0 0 1]  FollAlignAxisA=+X  BaseAlignAxisA=+Y  FollAlignAxisB=+Y  BaseAlignAxisB=+Z  RotationSequenceAxes=FollowerAxes  RotationSequence=XYX  RotationSequenceAngles=[0 0 0]  RotationSequenceAnglesUnits=deg  RotationMatrix=[1 0 0; 0 1 0; 0 0 1]
  Rigid Transform4 : sm_lib/Frames and Transforms/Rigid Transform  TranslationMethod=StandardAxis  TranslationStandardOffset=L3y/2  TranslationLengthUnit=m  TranslationStandardAxis=+Y  TranslationCartesianOffset=[0 0 0]  TranslationROffset=0  TranslationROffsetUnits=m  TranslationZOffset=0  TranslationZOffsetUnits=m  TranslationThetaOffset=0  TranslationThetaOffsetUnits=deg  RotationMethod=None  RotationAngleUnits=deg  RotationStandardAxis=+Z  RotationAngle=0.0  RotationArbitraryAxis=[0 0 1]  FollAlignAxisA=+X  BaseAlignAxisA=+Y  FollAlignAxisB=+Y  BaseAlignAxisB=+Z  RotationSequenceAxes=FollowerAxes  RotationSequence=XYX  RotationSequenceAngles=[0 0 0]  RotationSequenceAnglesUnits=deg  RotationMatrix=[1 0 0; 0 1 0; 0 0 1]
  Rigid Transform5 : sm_lib/Frames and Transforms/Rigid Transform  TranslationMethod=StandardAxis  TranslationStandardOffset=Hz/2  TranslationLengthUnit=m  TranslationStandardAxis=-Z  TranslationCartesianOffset=[0 0 0]  TranslationROffset=0  TranslationROffsetUnits=m  TranslationZOffset=0  TranslationZOffsetUnits=m  TranslationThetaOffset=0  TranslationThetaOffsetUnits=deg  RotationMethod=None  RotationAngleUnits=deg  RotationStandardAxis=+Z  RotationAngle=0.0  RotationArbitraryAxis=[0 0 1]  FollAlignAxisA=+X  BaseAlignAxisA=+Y  FollAlignAxisB=+Y  BaseAlignAxisB=+Z  RotationSequenceAxes=FollowerAxes  RotationSequence=XYX  RotationSequenceAngles=[0 0 0]  RotationSequenceAnglesUnits=deg  RotationMatrix=[1 0 0; 0 1 0; 0 0 1]
  Rigid Transform6 : sm_lib/Frames and Transforms/Rigid Transform  TranslationMethod=StandardAxis  TranslationStandardOffset=Hz/2  TranslationLengthUnit=m  TranslationStandardAxis=+Z  TranslationCartesianOffset=[0 0 0]  TranslationROffset=0  TranslationROffsetUnits=m  TranslationZOffset=0  TranslationZOffsetUnits=m  TranslationThetaOffset=0  TranslationThetaOffsetUnits=deg  RotationMethod=None  RotationAngleUnits=deg  RotationStandardAxis=+Z  RotationAngle=0.0  RotationArbitraryAxis=[0 0 1]  FollAlignAxisA=+X  BaseAlignAxisA=+Y  FollAlignAxisB=+Y  BaseAlignAxisB=+Z  RotationSequenceAxes=FollowerAxes  RotationSequence=XYX  RotationSequenceAngles=[0 0 0]  RotationSequenceAnglesUnits=deg  RotationMatrix=[1 0 0; 0 1 0; 0 0 1]
  Rigid Transform7 : sm_lib/Frames and Transforms/Rigid Transform  TranslationMethod=StandardAxis  TranslationStandardOffset=L3y/2  TranslationLengthUnit=m  TranslationStandardAxis=+Y  TranslationCartesianOffset=[0 0 0]  TranslationROffset=0  TranslationROffsetUnits=m  TranslationZOffset=0  TranslationZOffsetUnits=m  TranslationThetaOffset=0  TranslationThetaOffsetUnits=deg  RotationMethod=None  RotationAngleUnits=deg  RotationStandardAxis=+Z  RotationAngle=0.0  RotationArbitraryAxis=[0 0 1]  FollAlignAxisA=+X  BaseAlignAxisA=+Y  FollAlignAxisB=+Y  BaseAlignAxisB=+Z  RotationSequenceAxes=FollowerAxes  RotationSequence=XYX  RotationSequenceAngles=[0 0 0]  RotationSequenceAnglesUnits=deg  RotationMatrix=[1 0 0; 0 1 0; 0 0 1]
  SM_ANGS : Scope  NumInputPorts=12
  Selector : Selector  InputPortWidth=4  IndexOptions=Index vector (dialog)  Indices=[4 1 2 3]  OutputSizes=1
  Simulink-PS Converter{,1..3} (4 alike) : nesl_utility/Simulink-PS Converter  PhysicalDomain=network_engine_domain  SubClassName=ps_input  LeftPortType=input  RightPortType=output  PseudoPeriodic=off  Frequencies=[]  NoiseDistribution=none  NoiseParameters=[]  Unit=N*m  AffineConversion=off  InputFiltering=off  SimscapeFilterOrder=1  InputFilterTimeConstant=0.001  UdotUserProvided=1
  Solver Configuration : nesl_utility/Solver Configuration  PhysicalDomain=network_engine_domain  SubClassName=solver  LeftPortType=input  RightPortType=generic  Accelerate=off  Tones=[]  Harmonics=[]  SimulateNoise=off  Profile=off  UseLocalSampling=off  EnableSwitchedLinearOptims=on  FrequencyDomain=off  UseCCode=off  RelTol=0.001  AbsTol=1e-06  MinStep=1e-09  ToWorkspace=off  RevertToSquareIcSolve=off  NumHomotopyIterations=100  PhasorMode=off  PhasorModeNumHarmonics=1  OverrideAbsTol=off  DoDC=off  ResidualTolerance=1e-09  UseLocalSolver=off  LocalSolverChoice=NE_TRAPEZOIDAL_ADVANCER  LocalSolverSampleTime=0.01  DoFixedCost=off  MaxNonlinIter=3  MaxModeIter=2  LinearAlgebra=Sparse  DelaysMemoryBudget=1024  AutomaticFiltering=off  FilteringTimeConstant=0.001
  TURNTABLE : sm_lib/Body Elements/Solid  InertiaType=CalculateFromGeometry  Mass=1  MassUnits=kg  CenterOfMass=[0 0 0]  CenterOfMassUnits=m  MomentsOfInertia=[1 1 1]  MomentsOfInertiaUnits=kg*m^2  ProductsOfInertia=[0 0 0]  ProductsOfInertiaUnits=kg*m^2  DensityBased=on  Density=1000  DensityUnits=kg/(m^3)  DoExposeReferenceFrame=on  SerializedFrames=<Frames/>  GraphicType=FromGeometry  MarkerShape=Sphere  MarkerSize=10  GraphicVisPropType=SimpleVisualProperties  GraphicDiffuseColor=[1.0 1.0 0.2]  GraphicSpecularColor=[0.5 0.5 0.5 1.0]  GraphicAmbientColor=[0.15 0.15 0.15 1.0]  GraphicEmissiveColor=[0.0 0.0 0.0 1.0]  GraphicShininess=75  GraphicOpacity=1.0  GeometryShape=Cylinder  RectangleSize=[1 1]  RectangleSizeUnits=m  BrickDimensions=[1 1 1]  BrickDimensionUnits=m  CylinderRadius=Rturn  CylinderRadiusUnits=m  CylinderLength=Hz  CylinderLengthUnits=m  SphereRadius=1  SphereRadiusUnits=m  EllipsoidRadii=[1 1 1]  EllipsoidRadiiUnits=m  ExtrusionCrossSection=[1 1; -1 1; -1 -1; 1 -1]  ExtrusionCrossSectionUnits=m  ExtrusionLength=1  ExtrusionLengthUnits=m  PolygonNumSides=3  PolygonOuterRadius=1  PolygonOuterRadiusUnits=m  ExtGeomFileType=STEP  ExtGeomFileUnits=m  RevolutionCrossSection=[1 1; 1 -1; 2 -1; 2 1]  RevolutionCrossSectionUnits=m  RevolutionExtent=Full  RevolutionAngle=180  RevolutionAngleUnits=deg
  World Frame : sm_lib/Frames and Transforms/World Frame
  MODEL_BUS : Outport
  wires:
  [SM_BUS] -> MODEL_BUS/1
  [TH2_D] -> Create_SM_BUS/5(TH2_D)
  [TH1_D] -> Create_SM_BUS/2(TH1_D)
  [TH2_DD] -> Create_SM_BUS/4(TH2_DD)
  [TH2] -> Create_SM_BUS/6(TH2)
  [TH1_DD] -> Create_SM_BUS/3(TH1_DD)
  [TH1] -> Create_SM_BUS/1(TH1)
  Create_SM_BUS/1(SM_BUS) -> [SM_BUS]
  Bus Selector/2 -> SM_ANGS/2  "<TH1_D>"
  Bus Selector/3 -> SM_ANGS/3  "<TH1_DD>"
  Bus Selector/1 -> SM_ANGS/1  "<TH1>"
  Bus Selector/4 -> SM_ANGS/4  "<TH2>"
  Bus Selector/5 -> SM_ANGS/5  "<TH2_D>"
  Bus Selector/6 -> SM_ANGS/6  "<TH2_DD>"
  Bus Selector/7 -> SM_ANGS/7  "<TH3>"
  Bus Selector/8 -> SM_ANGS/8  "<TH3_D>"
  Bus Selector/9 -> SM_ANGS/9  "<TH3_DD>"
  [TH3_DD] -> Create_SM_BUS/7(TH3_DD)
  [TH3_D] -> Create_SM_BUS/8(TH3_D)
  [TH3] -> Create_SM_BUS/9(TH3)
  PS-Simulink Converter/1 -> [TH1]  "TH1"
  PS-Simulink Converter2/1 -> [TH1_DD]  "TH1_DD"
  PS-Simulink Converter1/1 -> [TH1_D]  "TH1_D"
  PS-Simulink Converter4/1 -> [TH2]  "TH2"
  PS-Simulink Converter6/1 -> [TH2_DD]  "TH2_DD"
  PS-Simulink Converter5/1 -> [TH2_D]  "TH2_D"
  PS-Simulink Converter3/1 -> [TH3]  "TH3"
  PS-Simulink Converter8/1 -> [TH3_DD]  "TH3_DD"
  PS-Simulink Converter7/1 -> [TH3_D]  "TH3_D"
  PS-Simulink Converter9/1 -> [TH4]  "TH4"
  PS-Simulink Converter11/1 -> [TH4_DD]  "TH4_DD"
  PS-Simulink Converter10/1 -> [TH4_D]  "TH4_D"
  [TH4_DD] -> Create_SM_BUS/10(TH4_DD)
  [TH4_D] -> Create_SM_BUS/11(TH4_D)
  [TH4] -> Create_SM_BUS/12(TH4)
  Bus Selector/12 -> SM_ANGS/12  "<TH4_DD>"
  Bus Selector/11 -> SM_ANGS/11  "<TH4_D>"
  Bus Selector/10 -> SM_ANGS/10  "<TH4>"
  [SM_BUS] -> Bus Selector/1
  Demux/1 -> Simulink-PS Converter/1
  Demux/2 -> Simulink-PS Converter1/1
  Demux/3 -> Simulink-PS Converter2/1
  Demux/4 -> Simulink-PS Converter3/1
  TQ_VEC/1 -> Reshape/1
  Selector/1 -> Demux/1
  Reshape/1 -> Selector/1
  connections:
  World Frame/RConn1 -- RJ_TURN/LConn1 -- Mechanism Configuration/RConn1 -- Solver Configuration/RConn1
  PS-Simulink Converter1/LConn1 -- RJ_TH1/RConn3
  PS-Simulink Converter2/LConn1 -- RJ_TH1/RConn4
  PS-Simulink Converter/LConn1 -- RJ_TH1/RConn2
  Rigid Transform5/LConn1 -- RJ_TURN/RConn1
  Rigid Transform5/RConn1 -- Rigid Transform6/LConn1 -- TURNTABLE/RConn1
  LocY2RZ/LConn1 -- Rigid Transform6/RConn1
  LocY2RZ/RConn1 -- RJ_TH1/LConn1
  Rigid Transform1/LConn1 -- LINK_1/RConn1 -- Rigid Transform/RConn1
  LocY2RZ2/LConn1 -- Rigid Transform1/RConn1
  LocY2RZ2/RConn1 -- RJ_TH2/LConn1
  RZ2LOCY1/LConn1 -- RJ_TH2/RConn1
  Rigid Transform2/RConn1 -- Rigid Transform3/LConn1 -- LINK_2/RConn1
  LocY2RZ4/LConn1 -- Rigid Transform3/RConn1
  RJ_TH1/RConn1 -- RZ2LOCY/LConn1
  RZ2LOCY/RConn1 -- Rigid Transform/LConn1
  RZ2LOCY1/RConn1 -- Rigid Transform2/LConn1
  RJ_TH3/LConn1 -- LocY2RZ4/RConn1
  LINK_3/RConn1 -- Rigid Transform7/LConn1 -- Rigid Transform4/RConn1
  LocY2RZ1/LConn1 -- Rigid Transform7/RConn1
  RZ2LOCY2/RConn1 -- Rigid Transform4/LConn1
  RZ2LOCY2/LConn1 -- RJ_TH3/RConn1
  RJ_TH2/RConn3 -- PS-Simulink Converter5/LConn1
  RJ_TH2/RConn2 -- PS-Simulink Converter4/LConn1
  RJ_TH2/RConn4 -- PS-Simulink Converter6/LConn1
  PS-Simulink Converter3/LConn1 -- RJ_TH3/RConn2
  RJ_TH3/RConn3 -- PS-Simulink Converter7/LConn1
  RJ_TH3/RConn4 -- PS-Simulink Converter8/LConn1
  RJ_TURN/RConn4 -- PS-Simulink Converter11/LConn1
  RJ_TURN/RConn3 -- PS-Simulink Converter10/LConn1
  RJ_TURN/RConn2 -- PS-Simulink Converter9/LConn1
  Simulink-PS Converter/RConn1 -- RJ_TURN/LConn2
  Simulink-PS Converter2/RConn1 -- RJ_TH2/LConn2
  Simulink-PS Converter3/RConn1 -- RJ_TH3/LConn2
  Simulink-PS Converter1/RConn1 -- RJ_TH1/LConn2

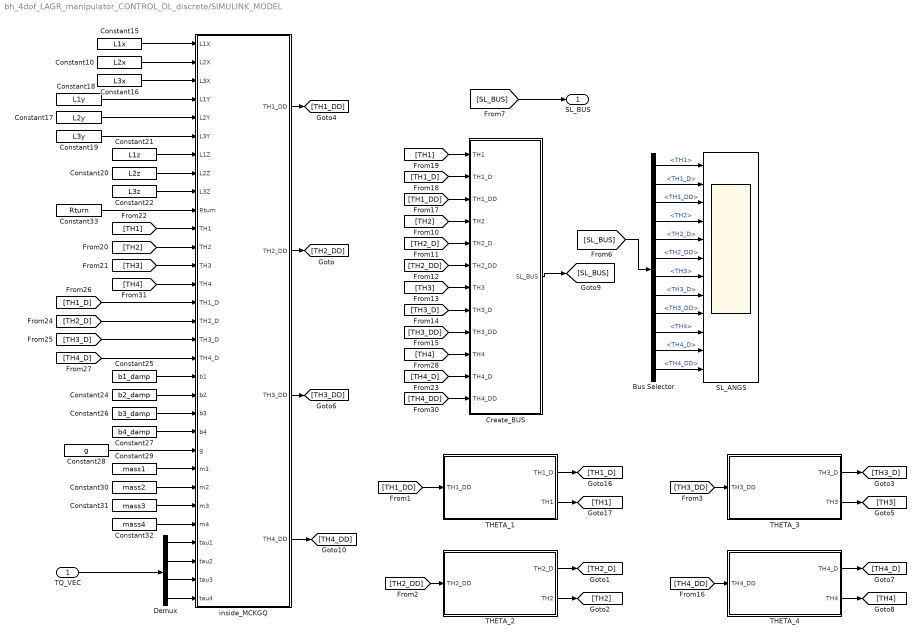
== system bh_4dof_LAGR_manipulator_CONTROL_DL_discrete/SIMULINK_MODEL ==
  TQ_VEC : Inport
  Bus Selector : BusSelector  OutputSignals=TH1,TH1_D,TH1_DD,TH2,TH2_D,TH2_DD,TH3,TH3_D,TH3_DD,TH4,TH4_D,TH4_DD
  Constant10 : Constant  Value=L2x
  Constant15 : Constant  Value=L1x
  Constant16 : Constant  Value=L3x
  Constant17 : Constant  Value=L2y
  Constant18 : Constant  Value=L1y
  Constant19 : Constant  Value=L3y
  Constant20 : Constant  Value=L2z
  Constant21 : Constant  Value=L1z
  Constant22 : Constant  Value=L3z
  Constant24 : Constant  Value=b2_damp
  Constant25 : Constant  Value=b1_damp
  Constant26 : Constant  Value=b3_damp
  Constant27 : Constant  Value=b4_damp
  Constant28 : Constant  Value=g
  Constant29 : Constant  Value=mass1
  Constant30 : Constant  Value=mass2
  Constant31 : Constant  Value=mass3
  Constant32 : Constant  Value=mass4
  Constant33 : Constant  Value=Rturn
  Create_BUS : Subsystem
  Demux : Demux
  SL_ANGS : Scope  NumInputPorts=12
  THETA_1 : Subsystem
  THETA_2 : Subsystem
  THETA_3 : Subsystem
  THETA_4 : Subsystem
  inside_MCKGQ : Subsystem
  SL_BUS : Outport
  wires:
  [SL_BUS] -> Bus Selector/1
  [SL_BUS] -> SL_BUS/1
  Create_BUS/1(SL_BUS) -> [SL_BUS]
  Bus Selector/2 -> SL_ANGS/2  "<TH1_D>"
  Bus Selector/3 -> SL_ANGS/3  "<TH1_DD>"
  Bus Selector/1 -> SL_ANGS/1  "<TH1>"
  Bus Selector/4 -> SL_ANGS/4  "<TH2>"
  Bus Selector/5 -> SL_ANGS/5  "<TH2_D>"
  Bus Selector/6 -> SL_ANGS/6  "<TH2_DD>"
  Bus Selector/7 -> SL_ANGS/7  "<TH3>"
  Bus Selector/8 -> SL_ANGS/8  "<TH3_D>"
  Bus Selector/9 -> SL_ANGS/9  "<TH3_DD>"
  [TH2_DD] -> THETA_2/1(TH2_DD)
  THETA_2/2(TH2) -> [TH2]
  THETA_2/1(TH2_D) -> [TH2_D]
  [TH1_DD] -> THETA_1/1(TH1_DD)
  THETA_1/1(TH1_D) -> [TH1_D]
  THETA_1/2(TH1) -> [TH1]
  inside_MCKGQ/2(TH2_DD) -> [TH2_DD]
  [TH3_DD] -> THETA_3/1(TH3_DD)
  THETA_3/2(TH3) -> [TH3]
  THETA_3/1(TH3_D) -> [TH3_D]
  inside_MCKGQ/1(TH1_DD) -> [TH1_DD]
  inside_MCKGQ/3(TH3_DD) -> [TH3_DD]
  [TH3_DD] -> Create_BUS/9(TH3_DD)
  [TH1] -> Create_BUS/1(TH1)
  [TH1_D] -> Create_BUS/2(TH1_D)
  [TH1_DD] -> Create_BUS/3(TH1_DD)
  [TH2] -> Create_BUS/4(TH2)
  [TH2_D] -> Create_BUS/5(TH2_D)
  [TH2_DD] -> Create_BUS/6(TH2_DD)
  [TH3] -> Create_BUS/7(TH3)
  [TH3_D] -> Create_BUS/8(TH3_D)
  [TH4_DD] -> THETA_4/1(TH4_DD)
  THETA_4/2(TH4) -> [TH4]
  THETA_4/1(TH4_D) -> [TH4_D]
  [TH2] -> inside_MCKGQ/12(TH2)
  [TH3] -> inside_MCKGQ/13(TH3)
  [TH1] -> inside_MCKGQ/11(TH1)
  Constant10/1 -> inside_MCKGQ/2(L2X)
  Constant16/1 -> inside_MCKGQ/3(L3X)
  Constant15/1 -> inside_MCKGQ/1(L1X)
  Constant19/1 -> inside_MCKGQ/6(L3Y)
  Constant17/1 -> inside_MCKGQ/5(L2Y)
  Constant18/1 -> inside_MCKGQ/4(L1Y)
  Constant22/1 -> inside_MCKGQ/9(L3Z)
  Constant20/1 -> inside_MCKGQ/8(L2Z)
  Constant21/1 -> inside_MCKGQ/7(L1Z)
  [TH1_D] -> inside_MCKGQ/15(TH1_D)
  [TH2_D] -> inside_MCKGQ/16(TH2_D)
  [TH3_D] -> inside_MCKGQ/17(TH3_D)
  [TH4_D] -> inside_MCKGQ/18(TH4_D)
  Constant25/1 -> inside_MCKGQ/19(b1)
  Constant24/1 -> inside_MCKGQ/20(b2)
  Constant26/1 -> inside_MCKGQ/21(b3)
  Constant27/1 -> inside_MCKGQ/22(b4)
  Constant28/1 -> inside_MCKGQ/23(g)
  Constant29/1 -> inside_MCKGQ/24(m1)
  Constant30/1 -> inside_MCKGQ/25(m2)
  Constant31/1 -> inside_MCKGQ/26(m3)
  Constant32/1 -> inside_MCKGQ/27(m4)
  Constant33/1 -> inside_MCKGQ/10(Rturn)
  [TH4_D] -> Create_BUS/11(TH4_D)
  [TH4_DD] -> Create_BUS/12(TH4_DD)
  [TH4] -> Create_BUS/10(TH4)
  [TH4] -> inside_MCKGQ/14(TH4)
  inside_MCKGQ/4(TH4_DD) -> [TH4_DD]
  Bus Selector/10 -> SL_ANGS/10  "<TH4>"
  Bus Selector/11 -> SL_ANGS/11  "<TH4_D>"
  Bus Selector/12 -> SL_ANGS/12  "<TH4_DD>"
  Demux/2 -> inside_MCKGQ/29(tau2)
  Demux/3 -> inside_MCKGQ/30(tau3)
  Demux/4 -> inside_MCKGQ/31(tau4)
  TQ_VEC/1 -> Demux/1
  Demux/1 -> inside_MCKGQ/28(tau1)

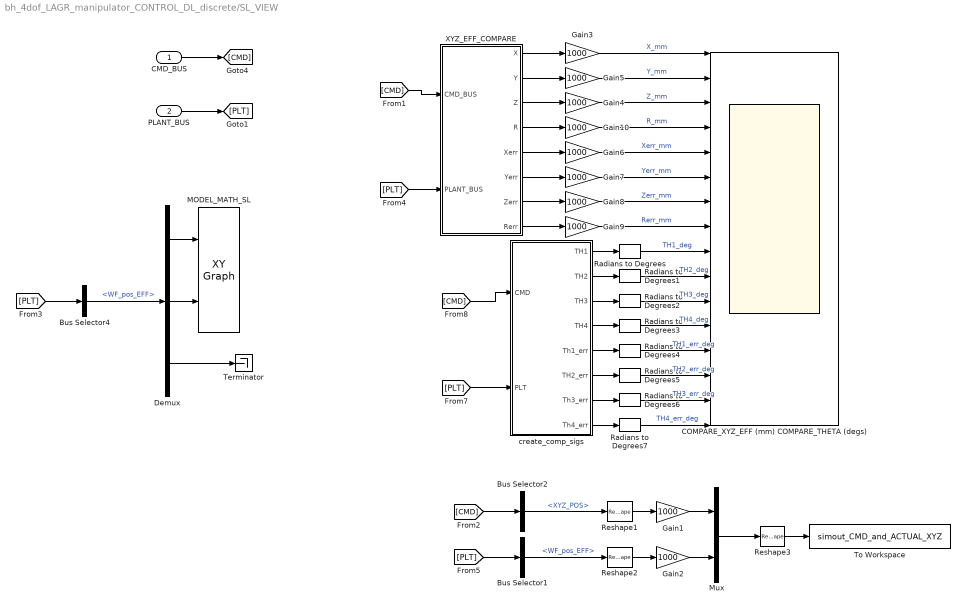
== system bh_4dof_LAGR_manipulator_CONTROL_DL_discrete/SL_VIEW ==
  CMD_BUS : Inport
  PLANT_BUS : Inport  Port=2
  Bus Selector1 : BusSelector  OutputSignals=CALC_POS_BUS.WF_pos_EFF
  Bus Selector2 : BusSelector  OutputSignals=XYZ_BUS.XYZ_POS
  Bus Selector4 : BusSelector  OutputSignals=CALC_POS_BUS.WF_pos_EFF
  COMPARE_XYZ_EFF (mm) COMPARE_THETA (degs) : Scope  NumInputPorts=16
  Demux : Demux  Outputs=3
  Gain{1..10} (10 alike) : Gain  Gain=1000
  MODEL_MATH_SL : simulink/Sinks/XY Graph  xmin=0  xmax=1.6  ymin=0  ymax=1.6  st=-1
  Mux : Mux  Inputs=2
  Radians to Degrees{,1..7} (8 alike) : simulink_extras/Transformations/Radians to Degrees
  Reshape1 : Reshape  OutputDimensionality=Column vector (2-D)
  Reshape2 : Reshape  OutputDimensionality=Column vector (2-D)
  Reshape3 : Reshape
  Terminator : Terminator
  To Workspace : ToWorkspace  VariableName=simout_CMD_and_ACTUAL_XYZ  SaveFormat=Structure With Time  SampleTime=0.001
  "XYZ_EFF_COMPARE " : Subsystem
  create_comp_sigs : Subsystem
  wires:
  CMD_BUS/1 -> [CMD]
  PLANT_BUS/1 -> [PLT]
  [CMD] -> "XYZ_EFF_COMPARE "/1(CMD_BUS)
  [PLT] -> "XYZ_EFF_COMPARE "/2(PLANT_BUS)
  "XYZ_EFF_COMPARE "/1(X) -> Gain3/1
  "XYZ_EFF_COMPARE "/2(Y) -> Gain5/1
  "XYZ_EFF_COMPARE "/3(Z) -> Gain4/1
  Gain3/1 -> COMPARE_XYZ_EFF (mm) COMPARE_THETA (degs)/1  "X_mm"
  Gain4/1 -> COMPARE_XYZ_EFF (mm) COMPARE_THETA (degs)/3  "Z_mm"
  Gain5/1 -> COMPARE_XYZ_EFF (mm) COMPARE_THETA (degs)/2  "Y_mm"
  Gain6/1 -> COMPARE_XYZ_EFF (mm) COMPARE_THETA (degs)/5  "Xerr_mm"
  Gain7/1 -> COMPARE_XYZ_EFF (mm) COMPARE_THETA (degs)/6  "Yerr_mm"
  Gain8/1 -> COMPARE_XYZ_EFF (mm) COMPARE_THETA (degs)/7  "Zerr_mm"
  "XYZ_EFF_COMPARE "/7(Zerr) -> Gain8/1
  "XYZ_EFF_COMPARE "/6(Yerr) -> Gain7/1
  "XYZ_EFF_COMPARE "/5(Xerr) -> Gain6/1
  [PLT] -> create_comp_sigs/2(PLT)
  [CMD] -> create_comp_sigs/1(CMD)
  create_comp_sigs/1(TH1) -> Radians to Degrees/1
  create_comp_sigs/2(TH2) -> Radians to Degrees1/1
  create_comp_sigs/3(TH3) -> Radians to Degrees2/1
  create_comp_sigs/4(TH4) -> Radians to Degrees3/1
  create_comp_sigs/5(Th1_err) -> Radians to Degrees4/1
  create_comp_sigs/6(TH2_err) -> Radians to Degrees5/1
  create_comp_sigs/7(Th3_err) -> Radians to Degrees6/1
  create_comp_sigs/8(Th4_err) -> Radians to Degrees7/1
  Radians to Degrees7/1 -> COMPARE_XYZ_EFF (mm) COMPARE_THETA (degs)/16  "TH4_err_deg"
  Radians to Degrees6/1 -> COMPARE_XYZ_EFF (mm) COMPARE_THETA (degs)/15  "TH3_err_deg"
  Radians to Degrees5/1 -> COMPARE_XYZ_EFF (mm) COMPARE_THETA (degs)/14  "TH2_err_deg"
  Radians to Degrees4/1 -> COMPARE_XYZ_EFF (mm) COMPARE_THETA (degs)/13  "TH1_err_deg"
  Radians to Degrees3/1 -> COMPARE_XYZ_EFF (mm) COMPARE_THETA (degs)/12  "TH4_deg"
  Radians to Degrees2/1 -> COMPARE_XYZ_EFF (mm) COMPARE_THETA (degs)/11  "TH3_deg"
  Radians to Degrees1/1 -> COMPARE_XYZ_EFF (mm) COMPARE_THETA (degs)/10  "TH2_deg"
  Radians to Degrees/1 -> COMPARE_XYZ_EFF (mm) COMPARE_THETA (degs)/9  "TH1_deg"
  Gain10/1 -> COMPARE_XYZ_EFF (mm) COMPARE_THETA (degs)/4  "R_mm"
  Gain9/1 -> COMPARE_XYZ_EFF (mm) COMPARE_THETA (degs)/8  "Rerr_mm"
  Bus Selector4/1 -> Demux/1  "<WF_pos_EFF>"
  Demux/1 -> MODEL_MATH_SL/1
  Demux/2 -> MODEL_MATH_SL/2
  [PLT] -> Bus Selector4/1
  Demux/3 -> Terminator/1
  [CMD] -> Bus Selector2/1
  [PLT] -> Bus Selector1/1
  Bus Selector2/1 -> Reshape1/1  "<XYZ_POS>"
  Bus Selector1/1 -> Reshape2/1  "<WF_pos_EFF>"
  Reshape2/1 -> Gain2/1
  Reshape1/1 -> Gain1/1
  Gain1/1 -> Mux/1
  Gain2/1 -> Mux/2
  Mux/1 -> Reshape3/1
  Reshape3/1 -> To Workspace/1
  "XYZ_EFF_COMPARE "/8(Rerr) -> Gain9/1
  "XYZ_EFF_COMPARE "/4(R) -> Gain10/1

== system bh_4dof_LAGR_manipulator_CONTROL_DL_discrete/SM_VIEW ==
  CMD_BUS : Inport
  PLANT_BUS : Inport  Port=2
  Bus Selector4 : BusSelector  OutputSignals=CALC_POS_BUS.WF_pos_EFF
  COMPARE_XYZ_EFF (mm) : Scope  NumInputPorts=3
  Demux : Demux  Outputs=3
  Gain : Gain  Gain=1000
  Gain1 : Gain  Gain=1000
  Gain2 : Gain  Gain=1000
  MODEL_MATH_SM : simulink/Sinks/XY Graph  xmin=0  xmax=1.6  ymin=0  ymax=1.6  st=-1
  PLANT_XYZ_EFF : Scope  NumInputPorts=3
  XYZ_EFF_COMPARE : Subsystem
  wires:
  CMD_BUS/1 -> [CMD]
  PLANT_BUS/1 -> [PLT]
  [CMD] -> XYZ_EFF_COMPARE/1(CMD_BUS)
  [PLT] -> XYZ_EFF_COMPARE/2(PLANT_BUS)
  XYZ_EFF_COMPARE/1(X) -> Gain/1
  XYZ_EFF_COMPARE/2(Y) -> Gain2/1
  XYZ_EFF_COMPARE/3(Z) -> Gain1/1
  Bus Selector4/1 -> Demux/1  "<WF_pos_EFF>"
  Demux/1 -> MODEL_MATH_SM/1, PLANT_XYZ_EFF/1
  Demux/2 -> MODEL_MATH_SM/2, PLANT_XYZ_EFF/2
  [PLT] -> Bus Selector4/1
  Demux/3 -> PLANT_XYZ_EFF/3
  Gain/1 -> COMPARE_XYZ_EFF (mm)/1
  Gain1/1 -> COMPARE_XYZ_EFF (mm)/3
  Gain2/1 -> COMPARE_XYZ_EFF (mm)/2
